simulink model "project_5"  (R2019a)
settings: Solver=VariableStepAuto  StartTime=0.0  StopTime=Sim_Time  RelTol=1e-3
values from neighbouring files (symbols this model uses):
  Cn = 2.3 * 3600    (= 8280)    [project_5_run.m]
  I = 2.3    [project_5_run.m]
  OCV = Data(:,2)    [project_5_run.m]
  R_c = Data(:,3)    [project_5_run.m]
  R_d = Data(:,4)    [project_5_run.m]
  SOC = Data(:,1)    [project_5_run.m]
settings Model: Creator=Nikita  LastModifiedBy=Nikita

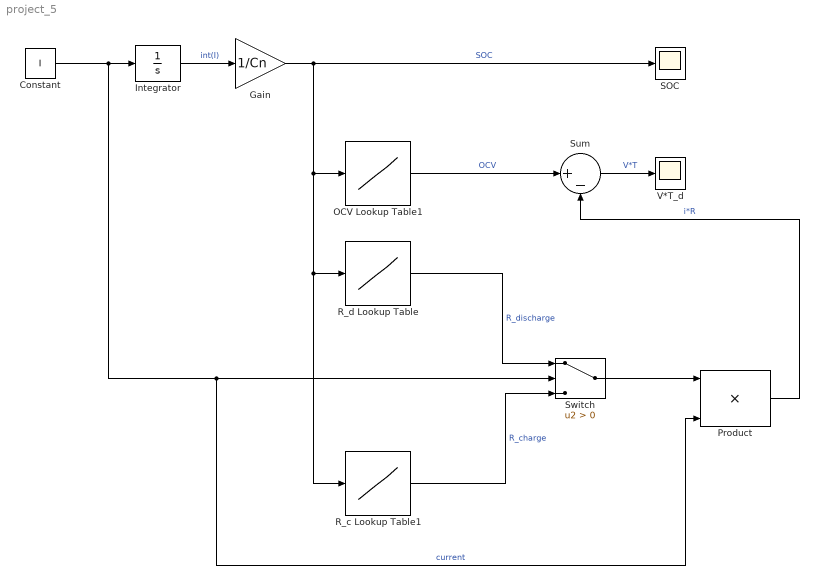
== system project_5 ==
  Constant : Constant  Value=I
  Gain : Gain  Gain=1/Cn
  Integrator : Integrator
  OCV Lookup Table1 : Lookup_n-D  NumberOfTableDimensions=1  BreakpointsForDimension1=SOC  Table=OCV  InternalRulePriority=Speed  RndMeth=Simplest  InputSameDT=on
  Product : Product  Inputs=3
  R_c Lookup Table1 : Lookup_n-D  NumberOfTableDimensions=1  BreakpointsForDimension1=SOC  Table=R_c  InternalRulePriority=Speed  RndMeth=Simplest  InputSameDT=on
  R_d Lookup Table : Lookup_n-D  NumberOfTableDimensions=1  BreakpointsForDimension1=SOC  Table=R_d  InternalRulePriority=Speed  RndMeth=Simplest  InputSameDT=on
  SOC : Scope
  Sum : Sum  Inputs=|+-
  Switch : Switch  Criteria=u2 > Threshold
  V*T_d : Scope
  wires:
  Constant/1 -> Product/3, Switch/2, Integrator/1  "current"
  Integrator/1 -> Gain/1  "int(I)"
  Gain/1 -> SOC/1, R_c Lookup Table1/1, R_d Lookup Table/1, OCV Lookup Table1/1  "SOC"
  OCV Lookup Table1/1 -> Sum/1  "OCV"
  R_d Lookup Table/1 -> Switch/1  "R_discharge"
  Product/1 -> Sum/2  "i*R"
  Sum/1 -> V*T_d/1  "V*T"
  R_c Lookup Table1/1 -> Switch/3  "R_charge"
  Switch/1 -> Product/1
